simulink model "Conventional"  (Simulink 10.1)
settings: Solver=ode4  StartTime=0  StopTime=endtime  FixedStep=0.1  MaxStep=0.05  RelTol=1e-5
values from neighbouring files (symbols this model uses):
  Av = 2.3*3.6    (= 8.28)    [InitiateCONVENTIONAL.m]
  Cd = 0.3    [InitiateCONVENTIONAL.m]
  Cr = 0.07    [InitiateCONVENTIONAL.m]
  DCT = 1    [InitiateCONVENTIONAL.m]
  Density = (85*19.6e6 + 15*32e6)/100    (= 21460000)    [InitiateCONVENTIONAL.m]
  Eta_gen = 0.6    [InitiateCONVENTIONAL.m]
  EtaGEAR = 0.97    [InitiateCONVENTIONAL.m]
  EtaICE = EtaICE_HeavyDIESEL    [InitiateCONVENTIONAL.m]
  grav = 9.81    [InitiateCONVENTIONAL.m]
  Mv = 10000    [InitiateCONVENTIONAL.m]
  Number_of_gears = 12    [InitiateCONVENTIONAL.m]
  Paux = Aux_vector(loop1)    [ConventionalBatch_2D.m]    (also in InitiateCONVENTIONAL.m = 3000)
  Pice_max = 400000    [InitiateCONVENTIONAL.m]
  PtoT = zeros(length(P),4)    [CreateICEmap.m]
  rho_air = 1.2    [InitiateCONVENTIONAL.m]
  rw = 0.90    (= 0.9)    [InitiateCONVENTIONAL.m]
  Tice_max = Pice_max/(wice_max*row/(length(EtaICE)-1))    [InitiateCONVENTIONAL.m]
  Utvx_vect = zeros(1,Number_of_gears+1)    [InitiateCONVENTIONAL.m]
  wice_max = 2500*2*pi/60    (= 261.799387799)    [InitiateCONVENTIONAL.m]
  wice_min = 700*2*pi/60    (= 73.3038285838)    [InitiateCONVENTIONAL.m]
undefined symbols (not defined in the file or in its folder): Tlim_ice, Wice
undefined symbols (not defined in the file): FuelConsICE, Tice
libraries: simulink_need_slupdate x1
settings Model: Creator=Mats  LastModifiedBy=ielmats  ExtModeTrigMode=oneshot  ExtModeArmWhenConnect=off
settings DataIOCC: SignalLoggingSaveFormat=ModelDataLogs  SignalLoggingName=sigsOut
settings OptimizationCC: BlockReduction=off  BooleanDataType=off  ExpressionDepthLimit=2147483647  InitFltsAndDblsToZero=on
settings DebuggingCC: ConsistencyChecking=warning  SaveWithParameterizedLinksMsg=none  SignalResolutionControl=TryResolveAllWithWarning  MultiTaskDSMMsg=warning  MultiTaskCondExecSysMsg=none  UnnecessaryDatatypeConvMsg=warning  FcnCallInpInsideContextMsg=warning  UnconnectedInputMsg=none  UnconnectedOutputMsg=none  UnconnectedLineMsg=none  StateNameClashWarn=warning  SFExecutionAtInitializationDiag=warning
settings HardwareCC: TargetUnknown=on

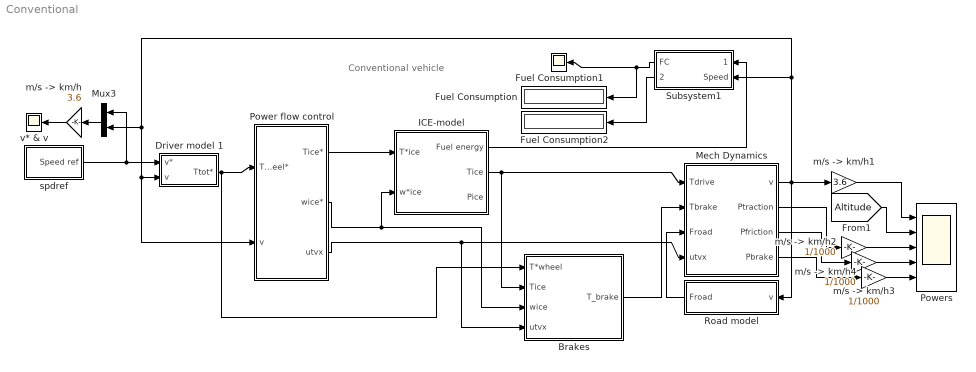
== system Conventional ==
  note: Conventional vehicle
  Brakes : Subsystem
  Driver model 1 : Subsystem  mask{Mv=Mv, rw=rw, Pmax=Pice_max*2}
      mask prompts: Mv "Vehicle Mass"; rw "Wheel Radius"; Pmax "Max Wheel Power"
      mask init:
      | Ti = 2 + 1*(Mv-1000)/19000;
      | Kv=4*Mv/Ti;
  Fuel Consumption : Display
  Fuel Consumption1 : Scope
  Fuel Consumption2 : Display
  ICE-model : Subsystem
  Mech Dynamics : Subsystem
  Mux3 : Mux  Inputs=2
  Power flow control : Subsystem
  Powers : Scope  NumInputPorts=5
  Road model : Subsystem
  Subsystem1 : Subsystem
  "m/s -> km/h" : Gain  Gain=3.6  SaturateOnIntegerOverflow=on  OutDataTypeStr=Inherit: Same as input  ParamDataTypeStr=Inherit: Same as input
  "m/s -> km/h1" : Gain  Gain=3.6  SaturateOnIntegerOverflow=on  OutDataTypeStr=Inherit: Same as input  ParamDataTypeStr=Inherit: Same as input
  "m/s -> km/h2" : Gain  Gain=1/1000  SaturateOnIntegerOverflow=on  OutDataTypeStr=Inherit: Same as input  ParamDataTypeStr=Inherit: Same as input
  "m/s -> km/h3" : Gain  Gain=1/1000  SaturateOnIntegerOverflow=on  OutDataTypeStr=Inherit: Same as input  ParamDataTypeStr=Inherit: Same as input
  "m/s -> km/h4" : Gain  Gain=1/1000  SaturateOnIntegerOverflow=on  OutDataTypeStr=Inherit: Same as input  ParamDataTypeStr=Inherit: Same as input
  spdref : Subsystem
  v* & v : Scope
  wires:
  ICE-model/2(Tice) -> Mech Dynamics/1(Tdrive), Brakes/2(Tice)
  spdref/1(Speed ref) -> Mux3/1, Driver model 1/1(v*)
  Driver model 1/1(Ttot*) -> Power flow control/1(Twheel*), Brakes/1(T*wheel)
  Mux3/1 -> "m/s -> km/h"/1
  Power flow control/1(Tice*) -> ICE-model/1(T*ice)
  Mech Dynamics/1(v) -> Road model/1("v "), Subsystem1/2(Speed), Driver model 1/2(v), Power flow control/2(v), Mux3/2, "m/s -> km/h1"/1
  Road model/1(Froad) -> Mech Dynamics/3(Froad)
  Brakes/1(T_brake) -> Mech Dynamics/2(Tbrake)
  ICE-model/1(Fuel energy) -> Subsystem1/1(Fuel energy)
  "m/s -> km/h"/1 -> v* & v/1
  Power flow control/2(wice*) -> Brakes/3(wice), ICE-model/2(w*ice)
  [Altitude] -> Powers/2
  Mech Dynamics/2(Ptraction) -> "m/s -> km/h2"/1
  Mech Dynamics/3(Pfriction) -> "m/s -> km/h3"/1
  Mech Dynamics/4(Pbrake) -> "m/s -> km/h4"/1
  "m/s -> km/h1"/1 -> Powers/1
  Power flow control/3(utvx) -> Mech Dynamics/4(utvx), Brakes/4(utvx)
  "m/s -> km/h2"/1 -> Powers/3
  "m/s -> km/h3"/1 -> Powers/4
  "m/s -> km/h4"/1 -> Powers/5
  Subsystem1/1(FC) -> Fuel Consumption/1, Fuel Consumption1/1
  Subsystem1/2(dist (mil)) -> Fuel Consumption2/1

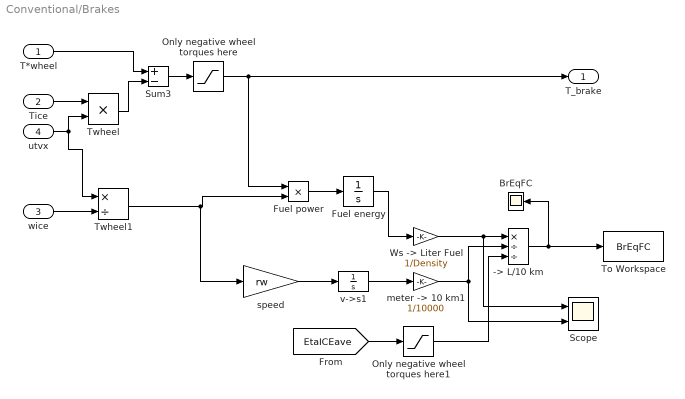
== system Conventional/Brakes ==
  T*wheel : Inport
  Tice : Inport  Port=2
  wice : Inport  Port=3
  utvx : Inport  Port=4
  -> L/10 km : Product  Inputs=*//  InputSameDT=on  SaturateOnIntegerOverflow=on  OutDataTypeStr=Inherit: Same as first input
  BrEqFC : Scope
  "Fuel energy " : Integrator
  Fuel power : Product  Inputs=**  InputSameDT=on  SaturateOnIntegerOverflow=on  OutDataTypeStr=Inherit: Same as first input
  Only negative wheel torques here : Saturate  UpperLimit=0  LowerLimit=-inf
  Only negative wheel torques here1 : Saturate  UpperLimit=inf  LowerLimit=eps
  Scope : Scope  NumInputPorts=2
  Sum3 : Sum  Inputs=+-  InputSameDT=on  SaturateOnIntegerOverflow=on  OutDataTypeStr=Inherit: Same as first input
  To Workspace : ToWorkspace  VariableName=BrEqFC  SampleTime=-1
  Twheel : Product  InputSameDT=on  SaturateOnIntegerOverflow=on  OutDataTypeStr=Inherit: Same as first input
  Twheel1 : Product  Inputs=*/  InputSameDT=on  SaturateOnIntegerOverflow=on  OutDataTypeStr=Inherit: Same as first input
  "Ws -> Liter Fuel" : Gain  Gain=1/Density  SaturateOnIntegerOverflow=on  OutDataTypeStr=Inherit: Same as input  ParamDataTypeStr=Inherit: Same as input
  "meter -> 10 km1" : Gain  Gain=1/10000  SaturateOnIntegerOverflow=on  OutDataTypeStr=Inherit: Same as input  ParamDataTypeStr=Inherit: Same as input
  speed : Gain  Gain=rw  SaturateOnIntegerOverflow=on  OutDataTypeStr=Inherit: Same as input  ParamDataTypeStr=Inherit: Same as input
  v->s1 : Integrator  InitialCondition=100  LimitOutput=on  LowerSaturationLimit=100
  T_brake : Outport  InitialOutput=0  VectorParamsAs1DForOutWhenUnconnected=off
  wires:
  Sum3/1 -> Only negative wheel torques here/1
  T*wheel/1 -> Sum3/1
  Only negative wheel torques here/1 -> T_brake/1, Fuel power/1
  v->s1/1 -> "meter -> 10 km1"/1
  speed/1 -> v->s1/1
  "Fuel energy "/1 -> "Ws -> Liter Fuel"/1
  Fuel power/1 -> "Fuel energy "/1
  "Ws -> Liter Fuel"/1 -> -> L/10 km/1, Scope/1
  "meter -> 10 km1"/1 -> -> L/10 km/2, Scope/2
  utvx/1 -> Twheel1/1, Twheel/2
  Tice/1 -> Twheel/1
  Twheel/1 -> Sum3/2
  [EtaICEave] -> Only negative wheel torques here1/1
  -> L/10 km/1 -> To Workspace/1, BrEqFC/1
  Only negative wheel torques here1/1 -> -> L/10 km/3
  Twheel1/1 -> speed/1, Fuel power/2
  wice/1 -> Twheel1/2

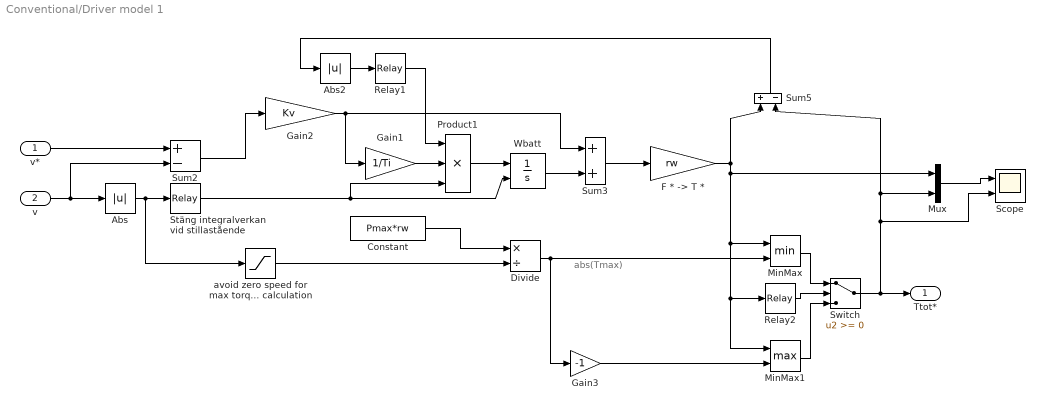
== system Conventional/Driver model 1 ==
  note: abs(Tmax)
  v* : Inport
  v : Inport  Port=2
  Abs : Abs  SaturateOnIntegerOverflow=on
  Abs2 : Abs  SaturateOnIntegerOverflow=on
  Constant : Constant  Value=Pmax*rw
  Divide : Product  Inputs=*/
  "F * -> T *" : Gain  Gain=rw  SaturateOnIntegerOverflow=on  OutDataTypeStr=Inherit: Same as input  ParamDataTypeStr=Inherit: Same as input
  Gain1 : Gain  Gain=1/Ti  SaturateOnIntegerOverflow=on  OutDataTypeStr=Inherit: Same as input  ParamDataTypeStr=Inherit: Same as input
  Gain2 : Gain  Gain=Kv  SaturateOnIntegerOverflow=on  OutDataTypeStr=Inherit: Same as input  ParamDataTypeStr=Inherit: Same as input
  Gain3 : Gain  Gain=-1  SaturateOnIntegerOverflow=on  OutDataTypeStr=Inherit: Same as input  ParamDataTypeStr=Inherit: Same as input
  MinMax : MinMax  Inputs=2
  MinMax1 : MinMax  Function=max  Inputs=2
  Mux : Mux  Inputs=2
  Product1 : Product  Inputs=3  InputSameDT=on  SaturateOnIntegerOverflow=on  OutDataTypeStr=Inherit: Same as first input
  Relay1 : Relay  OnOutputValue=0  OffOutputValue=1
  Relay2 : Relay  OnOutputValue=10  OffOutputValue=1
  Scope : Scope  NumInputPorts=2
  Stäng integralverkan vid stillastående : Relay  OnSwitchValue=0.3  OffSwitchValue=0.3-eps
  Sum2 : Sum  Inputs=+-  InputSameDT=on  SaturateOnIntegerOverflow=on  OutDataTypeStr=Inherit: Same as first input
  Sum3 : Sum  InputSameDT=on  SaturateOnIntegerOverflow=on  OutDataTypeStr=Inherit: Same as first input
  Sum5 : Sum  Inputs=+-  InputSameDT=on  SaturateOnIntegerOverflow=on  OutDataTypeStr=Inherit: Same as first input
  Switch : Switch
  Wbatt : Integrator  ExternalReset=falling  UpperSaturationLimit=1000  LowerSaturationLimit=-10000
  avoid zero speed for max torque calculation : Saturate  UpperLimit=inf  LowerLimit=5/3.6
  Ttot* : Outport  InitialOutput=0  VectorParamsAs1DForOutWhenUnconnected=off
  wires:
  Sum5/1 -> Abs2/1
  Relay1/1 -> Product1/1
  Abs2/1 -> Relay1/1
  Gain1/1 -> Product1/2
  Abs/1 -> Stäng integralverkan vid stillastående/1, avoid zero speed for max torque calculation/1
  Product1/1 -> Wbatt/1
  Sum3/1 -> "F * -> T *"/1
  Wbatt/1 -> Sum3/2
  "F * -> T *"/1 -> Mux/1, MinMax/1, MinMax1/1, Relay2/1, Sum5/1
  Gain2/1 -> Gain1/1, Sum3/1
  Stäng integralverkan vid stillastående/1 -> Product1/3, Wbatt/2
  Sum2/1 -> Gain2/1
  v*/1 -> Sum2/1
  v/1 -> Abs/1, Sum2/2
  Constant/1 -> Divide/1
  avoid zero speed for max torque calculation/1 -> Divide/2
  Divide/1 -> Gain3/1, MinMax/2
  Gain3/1 -> MinMax1/2
  Relay2/1 -> Switch/2
  MinMax/1 -> Switch/1
  MinMax1/1 -> Switch/3
  Switch/1 -> Ttot*/1, Scope/2, Mux/2, Sum5/2
  Mux/1 -> Scope/1

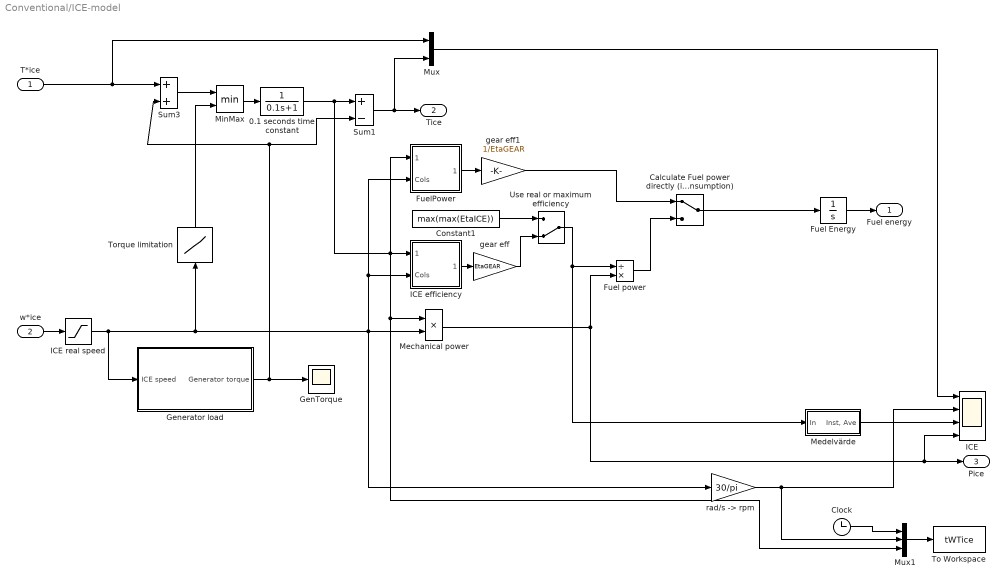
== system Conventional/ICE-model ==
  T*ice : Inport
  w*ice : Inport  Port=2
  0.1 seconds time constant : TransferFcn  Denominator=[0.1 1]
  Calculate Fuel power directly (including idle consumption) : ManualSwitch
  Clock : Clock
  Constant1 : Constant  Value=max(max(EtaICE))
  Fuel Energy : Integrator
  Fuel power : Product  Inputs=/*  InputSameDT=on  SaturateOnIntegerOverflow=on  OutDataTypeStr=Inherit: Same as first input
  FuelPower : Subsystem  mask(Lookup Table (2-D)){x=Tice, y=Wice, t=FuelConsICE}
      mask prompts: x "Row:"; y "Column:"; t "Table:"
      mask help: Performs 2-D linear interpolation of input values using the specified input/output table. Extrapolation is performed outside the table boundaries. The first dimension corresponds to the top (or left) input port.
      mask init:
      | [r,c]=size(t);
      | xt=reshape(x,prod(size(x)),1);
      | xi=xt(:,ones(1,c));
      | minx=min(x); maxx=max(x);
      | mint=min(min(t)); maxt=max(max(t));
      mask Display: plot(double(xi),double(t),double([minx maxx]),double([mint mint]),double([minx minx]),double([mint maxt]))
  GenTorque : Scope
  Generator load : Subsystem
  ICE : Scope  NumInputPorts=4
  ICE efficiency : Subsystem  mask(Lookup Table (2-D)){x=Tice, y=Wice, t=EtaICE}
      mask prompts: x "Row:"; y "Column:"; t "Table:"
      mask help: Performs 2-D linear interpolation of input values using the specified input/output table. Extrapolation is performed outside the table boundaries. The first dimension corresponds to the top (or left) input port.
      mask init:
      | [r,c]=size(t);
      | xt=reshape(x,prod(size(x)),1);
      | xi=xt(:,ones(1,c));
      | minx=min(x); maxx=max(x);
      | mint=min(min(t)); maxt=max(max(t));
      mask Display: plot(double(xi),double(t),double([minx maxx]),double([mint mint]),double([minx minx]),double([mint maxt]))
  ICE real speed : Saturate  UpperLimit=wice_max  LowerLimit=wice_min
  Mechanical power : Product  InputSameDT=on  SaturateOnIntegerOverflow=on  OutDataTypeStr=Inherit: Same as first input
  Medelvärde : Subsystem
  MinMax : MinMax  Inputs=2  InputSameDT=on  SaturateOnIntegerOverflow=on
  Mux : Mux  Inputs=2
  Mux1 : Mux  Inputs=3
  Sum1 : Sum  Inputs=+-  SaturateOnIntegerOverflow=on
  Sum3 : Sum  SaturateOnIntegerOverflow=on
  To Workspace : ToWorkspace  VariableName=tWTice  SampleTime=-1
  Torque limitation : Lookup  InputValues=Wice  Table=Tlim_ice  SaturateOnIntegerOverflow=on
  Use real or maximum efficiency : ManualSwitch  CurrentSetting=0
  gear eff : Gain  Gain=EtaGEAR  SaturateOnIntegerOverflow=on  OutDataTypeStr=Inherit: Same as input  ParamDataTypeStr=Inherit: Same as input
  gear eff1 : Gain  Gain=1/EtaGEAR  SaturateOnIntegerOverflow=on  OutDataTypeStr=Inherit: Same as input  ParamDataTypeStr=Inherit: Same as input
  "rad/s -> rpm" : Gain  Gain=30/pi  SaturateOnIntegerOverflow=on  OutDataTypeStr=Inherit: Same as input  ParamDataTypeStr=Inherit: Same as input
  Fuel energy : Outport  InitialOutput=0  VectorParamsAs1DForOutWhenUnconnected=off
  Tice : Outport  Port=2  InitialOutput=0  VectorParamsAs1DForOutWhenUnconnected=off
  Pice : Outport  Port=3  InitialOutput=0  VectorParamsAs1DForOutWhenUnconnected=off
  wires:
  Mux/1 -> ICE/1
  MinMax/1 -> 0.1 seconds time constant/1
  Torque limitation/1 -> MinMax/2
  Medelvärde/1("Inst, Ave") -> ICE/3
  "rad/s -> rpm"/1 -> ICE/2, Mux1/2
  Fuel Energy/1 -> Fuel energy/1
  w*ice/1 -> ICE real speed/1
  ICE efficiency/1(Out1) -> gear eff/1
  Clock/1 -> Mux1/1
  Mux1/1 -> To Workspace/1
  Mechanical power/1 -> Fuel power/2, Pice/1, ICE/4
  Generator load/1(Generator torque) -> GenTorque/1, Sum3/2, Sum1/2
  Sum1/1 -> Tice/1, Mux/2
  T*ice/1 -> Sum3/1, Mux/1
  Sum3/1 -> MinMax/1
  0.1 seconds time constant/1 -> Sum1/1, ICE efficiency/1(Rows), Mechanical power/1, Mux1/3, FuelPower/1(Rows)
  Fuel power/1 -> Calculate Fuel power directly (including idle consumption)/2
  Calculate Fuel power directly (including idle consumption)/1 -> Fuel Energy/1
  FuelPower/1(Out1) -> gear eff1/1
  gear eff1/1 -> Calculate Fuel power directly (including idle consumption)/1
  Constant1/1 -> Use real or maximum efficiency/1
  gear eff/1 -> Use real or maximum efficiency/2
  Use real or maximum efficiency/1 -> Fuel power/1, Medelvärde/1(In)
  ICE real speed/1 -> Generator load/1(ICE speed), Torque limitation/1, FuelPower/2(Cols), ICE efficiency/2(Cols), Mechanical power/2, "rad/s -> rpm"/1

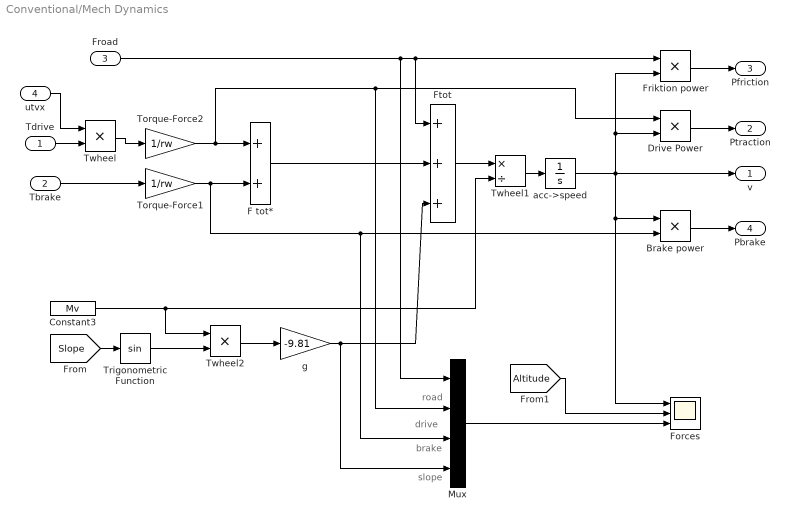
== system Conventional/Mech Dynamics ==
  note: road
  note: drive
  note: brake
  note: slope
  Tdrive : Inport
  Tbrake : Inport  Port=2
  Froad : Inport  Port=3
  utvx : Inport  Port=4
  Brake power : Product  InputSameDT=on  SaturateOnIntegerOverflow=on  OutDataTypeStr=Inherit: Same as first input
  Constant3 : Constant  Value=Mv
  Drive Power : Product  InputSameDT=on  SaturateOnIntegerOverflow=on  OutDataTypeStr=Inherit: Same as first input
  F tot* : Sum  InputSameDT=on  SaturateOnIntegerOverflow=on  OutDataTypeStr=Inherit: Same as first input
  Forces : Scope  NumInputPorts=3
  Friktion power : Product  InputSameDT=on  SaturateOnIntegerOverflow=on  OutDataTypeStr=Inherit: Same as first input
  Ftot : Sum  Inputs=+++  InputSameDT=on  SaturateOnIntegerOverflow=on  OutDataTypeStr=Inherit: Same as first input
  Mux : Mux
  Torque-Force1 : Gain  Gain=1/rw  SaturateOnIntegerOverflow=on  OutDataTypeStr=Inherit: Same as input  ParamDataTypeStr=Inherit: Same as input
  Torque-Force2 : Gain  Gain=1/rw  SaturateOnIntegerOverflow=on  OutDataTypeStr=Inherit: Same as input  ParamDataTypeStr=Inherit: Same as input
  Trigonometric Function : Trigonometry
  Twheel : Product  InputSameDT=on  SaturateOnIntegerOverflow=on  OutDataTypeStr=Inherit: Same as first input
  Twheel1 : Product  Inputs=*/  InputSameDT=on  SaturateOnIntegerOverflow=on  OutDataTypeStr=Inherit: Same as first input
  Twheel2 : Product  Inputs=**  InputSameDT=on  SaturateOnIntegerOverflow=on  OutDataTypeStr=Inherit: Same as first input
  acc->speed : Integrator  LimitOutput=on  LowerSaturationLimit=0
  g : Gain  Gain=-9.81  SaturateOnIntegerOverflow=on  OutDataTypeStr=Inherit: Same as input  ParamDataTypeStr=Inherit: Same as input
  v : Outport  InitialOutput=0  VectorParamsAs1DForOutWhenUnconnected=off
  Ptraction : Outport  Port=2  InitialOutput=0  VectorParamsAs1DForOutWhenUnconnected=off
  Pfriction : Outport  Port=3  InitialOutput=0  VectorParamsAs1DForOutWhenUnconnected=off
  Pbrake : Outport  Port=4  InitialOutput=0  VectorParamsAs1DForOutWhenUnconnected=off
  wires:
  Twheel1/1 -> acc->speed/1
  acc->speed/1 -> Friktion power/2, Drive Power/2, Brake power/1, Forces/1, v/1
  Tbrake/1 -> Torque-Force1/1
  F tot*/1 -> Ftot/2
  Ftot/1 -> Twheel1/1
  Froad/1 -> Ftot/1, Friktion power/1, Mux/1
  Friktion power/1 -> Pfriction/1
  Constant3/1 -> Twheel1/2, Twheel2/1
  Trigonometric Function/1 -> Twheel2/2
  Twheel2/1 -> g/1
  g/1 -> Ftot/3, Mux/4
  [Slope] -> Trigonometric Function/1
  [Altitude] -> Forces/2
  Mux/1 -> Forces/3
  Drive Power/1 -> Ptraction/1
  Torque-Force1/1 -> F tot*/2, Brake power/2, Mux/3
  Torque-Force2/1 -> F tot*/1, Drive Power/1, Mux/2
  Brake power/1 -> Pbrake/1
  Twheel/1 -> Torque-Force2/1
  Tdrive/1 -> Twheel/2
  utvx/1 -> Twheel/1

== system Conventional/Power flow control ==
  Twheel* : Inport
  v : Inport  Port=2
  For Starting : Saturate  UpperLimit=inf  LowerLimit=1/3.6
  Gear Selection : Subsystem
  Optimal operating point : Subsystem
  Scope : Scope  NumInputPorts=2
  Tractive Power : Product  InputSameDT=on  SaturateOnIntegerOverflow=on  OutDataTypeStr=Inherit: Same as first input
  "v -> w" : Gain  Gain=1/rw  SaturateOnIntegerOverflow=on  OutDataTypeStr=Inherit: Same as input  ParamDataTypeStr=Inherit: Same as input
  Tice* : Outport  VectorParamsAs1DForOutWhenUnconnected=off
  wice* : Outport  Port=2  VectorParamsAs1DForOutWhenUnconnected=off
  utvx : Outport  Port=3  VectorParamsAs1DForOutWhenUnconnected=off
  wires:
  "v -> w"/1 -> Gear Selection/1(w_wheel), For Starting/1
  Twheel*/1 -> Tractive Power/2
  v/1 -> "v -> w"/1, Scope/1
  Gear Selection/3(utvx) -> utvx/1
  Optimal operating point/2(wice*) -> Gear Selection/3(w_ice*)
  Optimal operating point/1(Tice*) -> Gear Selection/2(T_ice*)
  Tractive Power/1 -> Optimal operating point/1(P*), Scope/2
  Gear Selection/2(w*ice_new) -> wice*/1
  Gear Selection/1(T*ice_new) -> Tice*/1
  For Starting/1 -> Tractive Power/1

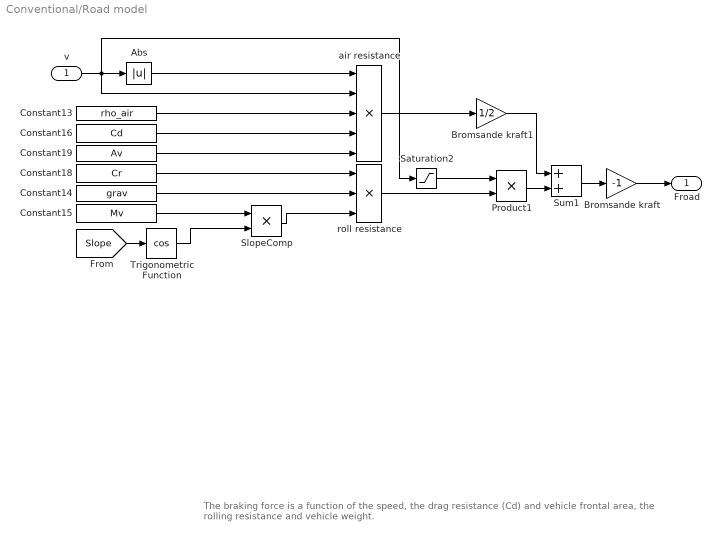
== system Conventional/Road model ==
  note: The braking force is  a function  of the speed, the drag resistance (Cd) and vehicle frontal area,
      | the rolling resistance and vehicle weight.
  "v " : Inport
  Abs : Abs  SaturateOnIntegerOverflow=on
  Bromsande kraft : Gain  Gain=-1  SaturateOnIntegerOverflow=on  OutDataTypeStr=Inherit: Same as input  ParamDataTypeStr=Inherit: Same as input
  Bromsande kraft1 : Gain  Gain=1/2  SaturateOnIntegerOverflow=on  OutDataTypeStr=Inherit: Same as input  ParamDataTypeStr=Inherit: Same as input
  Constant13 : Constant  Value=rho_air
  Constant14 : Constant  Value=grav
  Constant15 : Constant  Value=Mv
  Constant16 : Constant  Value=Cd
  Constant18 : Constant  Value=Cr
  Constant19 : Constant  Value=Av
  Product1 : Product  InputSameDT=on  SaturateOnIntegerOverflow=on  OutDataTypeStr=Inherit: Same as first input
  Saturation2 : Saturate  UpperLimit=1  LowerLimit=-1
  SlopeComp : Product  Inputs=**  InputSameDT=on  SaturateOnIntegerOverflow=on  OutDataTypeStr=Inherit: Same as first input
  Sum1 : Sum  InputSameDT=on  SaturateOnIntegerOverflow=on  OutDataTypeStr=Inherit: Same as first input
  Trigonometric Function : Trigonometry  Operator=cos
  air resistance : Product  Inputs=5  InputSameDT=on  SaturateOnIntegerOverflow=on  OutDataTypeStr=Inherit: Same as first input
  roll resistance : Product  Inputs=3  InputSameDT=on  SaturateOnIntegerOverflow=on  OutDataTypeStr=Inherit: Same as first input
  Froad : Outport  InitialOutput=0  VectorParamsAs1DForOutWhenUnconnected=off
  wires:
  Abs/1 -> air resistance/1
  Constant18/1 -> roll resistance/1
  Constant19/1 -> air resistance/5
  Constant16/1 -> air resistance/4
  Constant13/1 -> air resistance/3
  Product1/1 -> Sum1/2
  air resistance/1 -> Bromsande kraft1/1
  Saturation2/1 -> Product1/1
  Sum1/1 -> Bromsande kraft/1
  "v "/1 -> Abs/1, Saturation2/1, air resistance/2
  Bromsande kraft/1 -> Froad/1
  Bromsande kraft1/1 -> Sum1/1
  Trigonometric Function/1 -> SlopeComp/2
  SlopeComp/1 -> roll resistance/3
  [Slope] -> Trigonometric Function/1
  Constant14/1 -> roll resistance/2
  Constant15/1 -> SlopeComp/1
  roll resistance/1 -> Product1/2

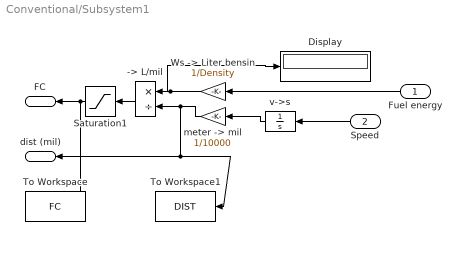
== system Conventional/Subsystem1 ==
  Fuel energy : Inport
  Speed : Inport  Port=2
  -> L/mil : Product  Inputs=*/  InputSameDT=on  SaturateOnIntegerOverflow=on  OutDataTypeStr=Inherit: Same as first input
  Display : Display
  Saturation1 : Saturate  UpperLimit=inf  LowerLimit=eps
  To Workspace : ToWorkspace  VariableName=FC  SampleTime=-1
  To Workspace1 : ToWorkspace  VariableName=DIST  SampleTime=-1
  "Ws -> Liter bensin" : Gain  Gain=1/Density  SaturateOnIntegerOverflow=on  OutDataTypeStr=Inherit: Same as input  ParamDataTypeStr=Inherit: Same as input
  "meter -> mil" : Gain  Gain=1/10000  SaturateOnIntegerOverflow=on  OutDataTypeStr=Inherit: Same as input  ParamDataTypeStr=Inherit: Same as input
  v->s : Integrator  InitialCondition=100  LimitOutput=on  LowerSaturationLimit=100
  FC : Outport  VectorParamsAs1DForOutWhenUnconnected=off
  dist (mil) : Outport  Port=2  VectorParamsAs1DForOutWhenUnconnected=off
  wires:
  "Ws -> Liter bensin"/1 -> Display/1, -> L/mil/1
  v->s/1 -> "meter -> mil"/1
  -> L/mil/1 -> Saturation1/1
  Speed/1 -> v->s/1
  Fuel energy/1 -> "Ws -> Liter bensin"/1
  Saturation1/1 -> FC/1, To Workspace/1
  "meter -> mil"/1 -> -> L/mil/2, To Workspace1/1, dist (mil)/1

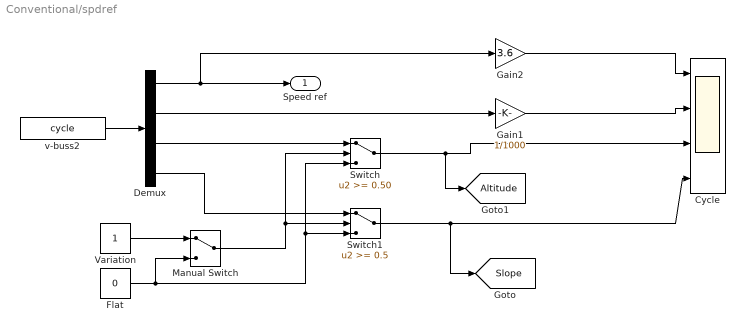
== system Conventional/spdref ==
  Cycle : Scope  NumInputPorts=4
  Demux : Demux
  Flat : Constant  Value=0
  Gain1 : Gain  Gain=1/1000  SaturateOnIntegerOverflow=on  OutDataTypeStr=Inherit: Same as input  ParamDataTypeStr=Inherit: Same as input
  Gain2 : Gain  Gain=3.6  SaturateOnIntegerOverflow=on  OutDataTypeStr=Inherit: Same as input  ParamDataTypeStr=Inherit: Same as input
  Manual Switch : ManualSwitch
  Switch : Switch  Threshold=0.50
  Switch1 : Switch  Threshold=0.5
  Variation : Constant
  v-buss2 : FromWorkspace  VariableName=cycle  SampleTime=.2  ZeroCross=off
  Speed ref : Outport  VectorParamsAs1DForOutWhenUnconnected=off
  tag scope: Altitude=global, Slope=global
  wires:
  v-buss2/1 -> Demux/1
  Demux/4 -> Switch1/1
  Demux/1 -> Speed ref/1, Gain2/1
  Demux/3 -> Switch/1
  Demux/2 -> Gain1/1
  Flat/1 -> Switch1/3, Switch/3, Manual Switch/2
  Switch/1 -> Cycle/3, [Altitude]
  Switch1/1 -> Cycle/4, [Slope]
  Variation/1 -> Manual Switch/1
  Manual Switch/1 -> Switch/2, Switch1/2
  Gain1/1 -> Cycle/2
  Gain2/1 -> Cycle/1

== system Conventional/ICE-model/FuelPower ==
  Rows : Inport
  Cols : Inport  Port=2
  Look-Up Table (2-D) : Lookup2D  RowIndex=x  ColumnIndex=y  Table=t  SaturateOnIntegerOverflow=on  InputSameDT=on
  Out1 : Outport  VectorParamsAs1DForOutWhenUnconnected=off
  wires:
  Look-Up Table (2-D)/1 -> Out1/1
  Cols/1 -> Look-Up Table (2-D)/2
  Rows/1 -> Look-Up Table (2-D)/1

== system Conventional/ICE-model/Generator load ==
  ICE speed : Inport
  Constant : Constant  Value=Paux
  Generator Efficiency : Constant  Value=Eta_gen
  Generator Mech Power : Product  Inputs=/*  InputSameDT=on  SaturateOnIntegerOverflow=on  OutDataTypeStr=Inherit: Same as first input
  Generator Mech Torque : Product  Inputs=/*  InputSameDT=on  SaturateOnIntegerOverflow=on  OutDataTypeStr=Inherit: Same as first input
  Saturation : Saturate  UpperLimit=Paux*2/(wice_max/5)  LowerLimit=0
  Generator torque : Outport  VectorParamsAs1DForOutWhenUnconnected=off
  wires:
  Constant/1 -> Generator Mech Power/2
  Generator Efficiency/1 -> Generator Mech Power/1
  Generator Mech Power/1 -> Generator Mech Torque/2
  ICE speed/1 -> Generator Mech Torque/1
  Generator Mech Torque/1 -> Saturation/1
  Saturation/1 -> Generator torque/1

== system Conventional/ICE-model/ICE efficiency ==
  Rows : Inport
  Cols : Inport  Port=2
  Look-Up Table (2-D) : Lookup2D  RowIndex=x  ColumnIndex=y  Table=t  SaturateOnIntegerOverflow=on  InputSameDT=on
  Out1 : Outport  VectorParamsAs1DForOutWhenUnconnected=off
  wires:
  Look-Up Table (2-D)/1 -> Out1/1
  Cols/1 -> Look-Up Table (2-D)/2
  Rows/1 -> Look-Up Table (2-D)/1

== system Conventional/ICE-model/Medelvärde ==
  note: Denna del "mäter" tiden då motorn
      | är till, d.v.s. då verkningsgraden är
      | större än 1 %. Om den är 5 % antas
      | motorn stå still.
  In : Inport
  Integral : Integrator
  Integral1 : Integrator  InitialCondition=4  LimitOutput=on  LowerSaturationLimit=1
  Medelv : Product  Inputs=*/  InputSameDT=on  SaturateOnIntegerOverflow=on  OutDataTypeStr=Inherit: Same as first input
  Medelv1 : Product  Inputs=**  InputSameDT=on  SaturateOnIntegerOverflow=on  OutDataTypeStr=Inherit: Same as first input
  Mux : Mux  Inputs=2
  Relay : Relay  OnSwitchValue=0.05  OffSwitchValue=0.04
  Scope : Scope
  "Inst, Ave" : Outport  VectorParamsAs1DForOutWhenUnconnected=off
  tag scope: EtaICEave=global
  wires:
  Mux/1 -> "Inst, Ave"/1
  Medelv/1 -> Mux/2, [EtaICEave], Scope/1
  Relay/1 -> Integral1/1, Medelv1/2
  In/1 -> Mux/1, Relay/1, Medelv1/1
  Integral/1 -> Medelv/1
  Integral1/1 -> Medelv/2
  Medelv1/1 -> Integral/1

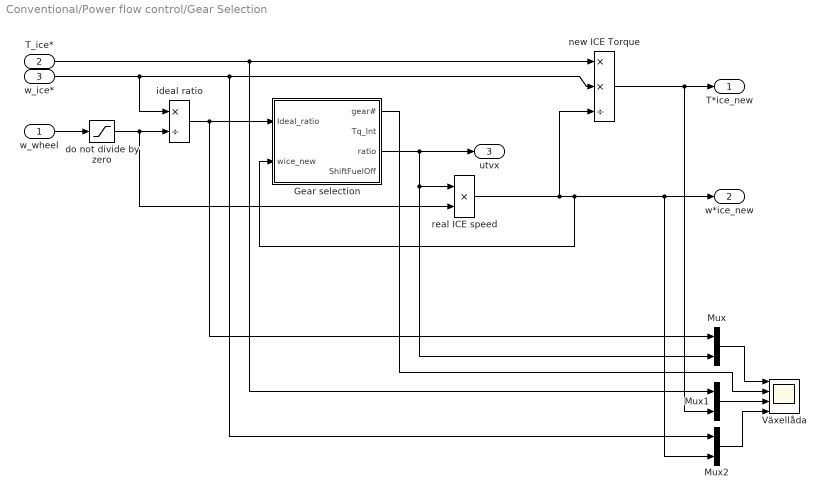
== system Conventional/Power flow control/Gear Selection ==
  w_wheel : Inport
  T_ice* : Inport  Port=2
  w_ice* : Inport  Port=3
  Gear selection : Subsystem
  Mux : Mux  Inputs=2
  Mux1 : Mux  Inputs=2
  Mux2 : Mux  Inputs=2
  Växellåda : Scope  NumInputPorts=4
  do not divide by zero : Saturate  UpperLimit=inf  LowerLimit=1
  ideal ratio : Product  Inputs=*/  InputSameDT=on  SaturateOnIntegerOverflow=on  OutDataTypeStr=Inherit: Same as first input
  new ICE Torque : Product  Inputs=**/  InputSameDT=on  SaturateOnIntegerOverflow=on  OutDataTypeStr=Inherit: Same as first input
  real ICE speed : Product  Inputs=**  InputSameDT=on  SaturateOnIntegerOverflow=on  OutDataTypeStr=Inherit: Same as first input
  T*ice_new : Outport  VectorParamsAs1DForOutWhenUnconnected=off
  w*ice_new : Outport  Port=2  VectorParamsAs1DForOutWhenUnconnected=off
  utvx : Outport  Port=3  VectorParamsAs1DForOutWhenUnconnected=off
  wires:
  w_ice*/1 -> ideal ratio/1, Mux2/1, new ICE Torque/2
  ideal ratio/1 -> Gear selection/1(Ideal_ratio), Mux/1
  real ICE speed/1 -> Gear selection/2(wice_new), w*ice_new/1, Mux2/2, new ICE Torque/3
  T_ice*/1 -> Mux1/1, new ICE Torque/1
  do not divide by zero/1 -> ideal ratio/2, real ICE speed/2
  w_wheel/1 -> do not divide by zero/1
  Mux/1 -> Växellåda/1
  Mux1/1 -> Växellåda/3
  Mux2/1 -> Växellåda/4
  Gear selection/3(ratio) -> real ICE speed/1, Mux/2, utvx/1
  Gear selection/1(gear#) -> Växellåda/2
  new ICE Torque/1 -> T*ice_new/1, Mux1/2

== system Conventional/Power flow control/Optimal operating point ==
  note: ICE'n antas
      | inte kunna
      | motorbromsa
  P* : Inport
  -> w : Product  Inputs=/*  InputSameDT=on  SaturateOnIntegerOverflow=on  OutDataTypeStr=Inherit: Same as first input
  -> w2 : Product  Inputs=/*  InputSameDT=on  SaturateOnIntegerOverflow=on  OutDataTypeStr=Inherit: Same as first input
  Saturation1 : Saturate  UpperLimit=Pice_max  LowerLimit=eps
  Saturation3 : Saturate  UpperLimit=Tice_max  LowerLimit=eps
  Saturation4 : Saturate  UpperLimit=wice_max  LowerLimit=wice_min
  Topt_ice : Lookup  InputValues=PtoT(:,1)  Table=PtoT(:,2)  SaturateOnIntegerOverflow=on
  Tice* : Outport  InitialOutput=0  VectorParamsAs1DForOutWhenUnconnected=off
  wice* : Outport  Port=2  InitialOutput=0  VectorParamsAs1DForOutWhenUnconnected=off
  wires:
  P*/1 -> Saturation1/1
  -> w/1 -> Saturation4/1
  Topt_ice/1 -> Saturation3/1
  Saturation1/1 -> Topt_ice/1, -> w/2, -> w2/2
  Saturation3/1 -> -> w/1
  Saturation4/1 -> wice*/1, -> w2/1
  -> w2/1 -> Tice*/1

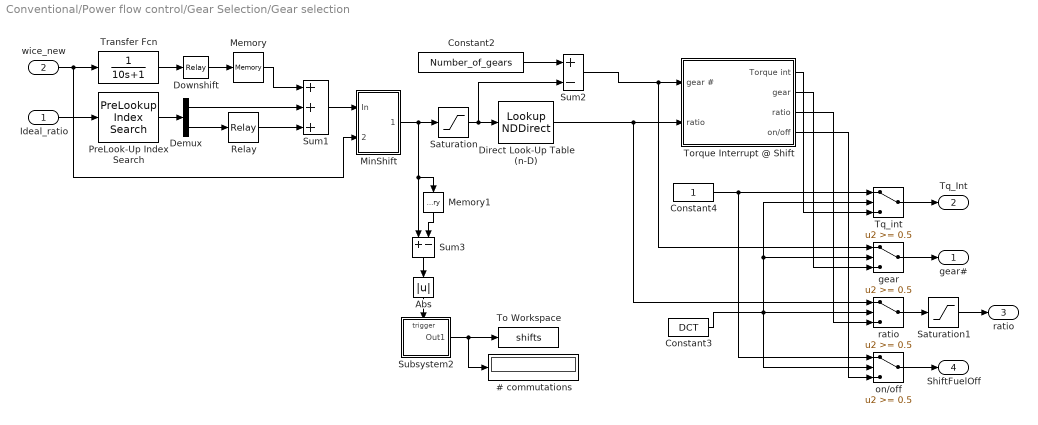
== system Conventional/Power flow control/Gear Selection/Gear selection ==
  Ideal_ratio : Inport
  wice_new : Inport  Port=2
  # commutations : Display
  Abs : Abs  SaturateOnIntegerOverflow=on
  Constant2 : Constant  Value=Number_of_gears
  Constant3 : Constant  Value=DCT
  Constant4 : Constant
  Demux : Demux  Outputs=2
      settings: DisplayOption=none
  Direct Look-Up Table (n-D) : LookupNDDirect  NumberOfTableDimensions=1  Table=Utvx_vect
  Downshift : Relay  OnSwitchValue=0.85*wice_max  OffSwitchValue=0.40*wice_max  OnOutputValue=0  OffOutputValue=Speedy
  Memory : Memory
  Memory1 : Memory
  MinShift : Subsystem
  PreLook-Up Index Search : simulink_need_slupdate/PreLookup Index Search  bpData=Utvx_vect  searchMode=Binary Search  cacheBpFlag=off  outputFlag=off  IndexDataType=uint32  extrapMode=Linear Extrapolation  rangeErrorMode=None
      settings: SourceProductBaseCode=SL
  Relay : Relay  OnSwitchValue=0.52  OffSwitchValue=0.48
  Saturation : Saturate  UpperLimit=Number_of_gears-1  LowerLimit=0
  Saturation1 : Saturate  UpperLimit=max(Utvx_vect)  LowerLimit=min(Utvx_vect)
  Subsystem2 : Subsystem  TreatAsAtomicUnit=on
  Sum1 : Sum  Inputs=+++  SaturateOnIntegerOverflow=on
  Sum2 : Sum  Inputs=+-  SaturateOnIntegerOverflow=on
  Sum3 : Sum  Inputs=+-  SaturateOnIntegerOverflow=on
  To Workspace : ToWorkspace  VariableName=shifts  SampleTime=-1
  Torque Interrupt @ Shift : Subsystem
  Tq_int : Switch  Threshold=0.5  SaturateOnIntegerOverflow=on
  Transfer Fcn : TransferFcn  Denominator=[10 1]
  "gear " : Switch  Threshold=0.5  SaturateOnIntegerOverflow=on
  "on/off " : Switch  Threshold=0.5  SaturateOnIntegerOverflow=on
  "ratio " : Switch  Threshold=0.5  SaturateOnIntegerOverflow=on
  gear# : Outport  VectorParamsAs1DForOutWhenUnconnected=off
  Tq_Int : Outport  Port=2  VectorParamsAs1DForOutWhenUnconnected=off
  ratio : Outport  Port=3  VectorParamsAs1DForOutWhenUnconnected=off
  ShiftFuelOff : Outport  Port=4  VectorParamsAs1DForOutWhenUnconnected=off
  wires:
  Ideal_ratio/1 -> PreLook-Up Index Search/1
  Memory/1 -> Sum1/1
  wice_new/1 -> Transfer Fcn/1, MinShift/2(Speed)
  Downshift/1 -> Memory/1
  Transfer Fcn/1 -> Downshift/1
  PreLook-Up Index Search/1 -> Demux/1
  Demux/2 -> Relay/1
  Relay/1 -> Sum1/3
  Demux/1 -> Sum1/2
  Direct Look-Up Table (n-D)/1 -> Torque Interrupt @ Shift/2(ratio), "ratio "/1
  Constant2/1 -> Sum2/1
  Sum2/1 -> Torque Interrupt @ Shift/1(gear #), "gear "/1
  Saturation/1 -> Sum2/2, Direct Look-Up Table (n-D)/1
  Torque Interrupt @ Shift/1(Torque int) -> Tq_int/3
  Torque Interrupt @ Shift/2(gear) -> "gear "/3
  Torque Interrupt @ Shift/4(on/off) -> "on/off "/3
  Torque Interrupt @ Shift/3("ratio ") -> "ratio "/3
  Constant3/1 -> Tq_int/2, "gear "/2, "ratio "/2, "on/off "/2
  Constant4/1 -> Tq_int/1, "on/off "/1
  Tq_int/1 -> Tq_Int/1
  "gear "/1 -> gear#/1
  "ratio "/1 -> Saturation1/1
  "on/off "/1 -> ShiftFuelOff/1
  Subsystem2/1(Out1) -> # commutations/1, To Workspace/1
  Memory1/1 -> Sum3/2
  Sum3/1 -> Abs/1
  Abs/1 -> Subsystem2/Trigger
  MinShift/1(Out) -> Sum3/1, Memory1/1, Saturation/1
  Sum1/1 -> MinShift/1(In)
  Saturation1/1 -> ratio/1

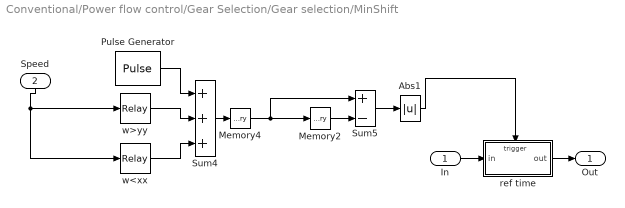
== system Conventional/Power flow control/Gear Selection/Gear selection/MinShift ==
  In : Inport
  Speed : Inport  Port=2
  Abs1 : Abs  SaturateOnIntegerOverflow=on
  Memory2 : Memory
  Memory4 : Memory
  Pulse Generator : DiscretePulseGenerator  Period=16  PulseWidth=8  SampleTime=0.2
  Sum4 : Sum  Inputs=+++  SaturateOnIntegerOverflow=on
  Sum5 : Sum  Inputs=+-  SaturateOnIntegerOverflow=on
  ref time : Subsystem  AncestorBlock=|  TreatAsAtomicUnit=on
      | simulink/Model-Wide
      | Utilities/Trigger-Based
      | Linearization
  w<xx : Relay  OnSwitchValue=wice_min*1.2  OffSwitchValue=wice_min*1.1  OnOutputValue=0  OffOutputValue=1
  w>yy : Relay  OnSwitchValue=wice_max*0.8  OffSwitchValue=wice_max*0.7
  Out : Outport  VectorParamsAs1DForOutWhenUnconnected=off
  wires:
  w>yy/1 -> Sum4/2
  w<xx/1 -> Sum4/3
  Pulse Generator/1 -> Sum4/1
  Sum4/1 -> Memory4/1
  Memory2/1 -> Sum5/2
  Sum5/1 -> Abs1/1
  Abs1/1 -> ref time/Trigger
  Memory4/1 -> Memory2/1, Sum5/1
  Speed/1 -> w>yy/1, w<xx/1
  In/1 -> ref time/1(in)
  ref time/1(out) -> Out/1

== system Conventional/Power flow control/Gear Selection/Gear selection/Subsystem2 ==
  Trigger : TriggerPort  TriggerType=either  VariantControl=Variant
  Constant : Constant
  Memory : Memory  InheritSampleTime=on
  Sum : Sum  InputSameDT=on  SaturateOnIntegerOverflow=on  OutDataTypeStr=Inherit: Same as first input
  Out1 : Outport  VectorParamsAs1DForOutWhenUnconnected=off
  wires:
  Sum/1 -> Memory/1, Out1/1
  Memory/1 -> Sum/2
  Constant/1 -> Sum/1

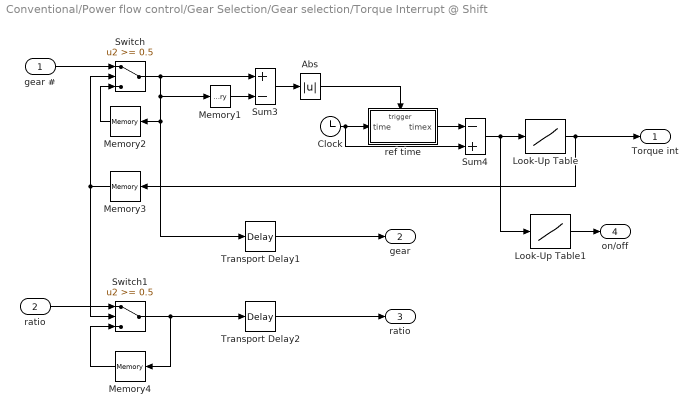
== system Conventional/Power flow control/Gear Selection/Gear selection/Torque Interrupt @ Shift ==
  gear # : Inport
  ratio : Inport  Port=2
  Abs : Abs  SaturateOnIntegerOverflow=on
  Clock : Clock
  Look-Up Table : Lookup  InputValues=[0 0.2 0.8 1.0]  Table=[1 0 0 1]  LookUpMeth=Interpolation-Use End Values  SaturateOnIntegerOverflow=on
  Look-Up Table1 : Lookup  InputValues=[0 0.2 0.2+eps 0.8-eps 0.8 1.0]  Table=[1 1 0 0 1 1]  LookUpMeth=Interpolation-Use End Values  SaturateOnIntegerOverflow=on
  Memory1 : Memory
  Memory2 : Memory  InheritSampleTime=on
  Memory3 : Memory  InheritSampleTime=on
  Memory4 : Memory  InheritSampleTime=on
  Sum3 : Sum  Inputs=+-  SaturateOnIntegerOverflow=on
  Sum4 : Sum  Inputs=-+  SaturateOnIntegerOverflow=on
  Switch : Switch  Threshold=0.5  SaturateOnIntegerOverflow=on
  Switch1 : Switch  Threshold=0.5  SaturateOnIntegerOverflow=on
  Transport Delay1 : TransportDelay  DelayTime=0.6
  Transport Delay2 : TransportDelay  DelayTime=0.6
  ref time : Subsystem  AncestorBlock=|  TreatAsAtomicUnit=on
      | simulink/Model-Wide
      | Utilities/Trigger-Based
      | Linearization
  Torque int : Outport  VectorParamsAs1DForOutWhenUnconnected=off
  gear : Outport  Port=2  VectorParamsAs1DForOutWhenUnconnected=off
  "ratio " : Outport  Port=3  VectorParamsAs1DForOutWhenUnconnected=off
  on/off : Outport  Port=4  VectorParamsAs1DForOutWhenUnconnected=off
  wires:
  Memory1/1 -> Sum3/2
  Sum3/1 -> Abs/1
  Abs/1 -> ref time/Trigger
  Clock/1 -> ref time/1(time), Sum4/2
  Sum4/1 -> Look-Up Table/1, Look-Up Table1/1
  ref time/1(timex) -> Sum4/1
  Look-Up Table/1 -> Torque int/1, Memory3/1
  gear #/1 -> Switch/1
  Switch/1 -> Sum3/1, Memory2/1, Transport Delay1/1, Memory1/1
  Transport Delay1/1 -> gear/1
  Memory2/1 -> Switch/3
  Memory3/1 -> Switch/2, Switch1/2
  ratio/1 -> Switch1/1
  Switch1/1 -> Memory4/1, Transport Delay2/1
  Memory4/1 -> Switch1/3
  Transport Delay2/1 -> "ratio "/1
  Look-Up Table1/1 -> on/off/1

== system Conventional/Power flow control/Gear Selection/Gear selection/MinShift/ref time ==
  in : Inport
  Trigger : TriggerPort  VariantControl=Variant
  Zero-Order Hold : ZeroOrderHold  SampleTime=-1
  out : Outport  VectorParamsAs1DForOutWhenUnconnected=off
  wires:
  in/1 -> Zero-Order Hold/1
  Zero-Order Hold/1 -> out/1

== system Conventional/Power flow control/Gear Selection/Gear selection/Torque Interrupt @ Shift/ref time ==
  time : Inport
  Trigger : TriggerPort  VariantControl=Variant
  Zero-Order Hold : ZeroOrderHold  SampleTime=-1
  timex : Outport  VectorParamsAs1DForOutWhenUnconnected=off
  wires:
  time/1 -> Zero-Order Hold/1
  Zero-Order Hold/1 -> timex/1
